simulink model "bicyclemodel_sin"  (R2021a)
settings: Solver=FixedStepAuto  StartTime=0.0  StopTime=tf  FixedStep=dt  RelTol=1e-3
values from neighbouring files (symbols this model uses):
  I = 2500    [E3_7.m]    (also in E3_8.m)
  Kf = 55000    [E3_7.m]    (also in E3_8.m = 72500)
  Kr = 60000    [E3_7.m]    (also in E3_8.m = 42500)
  lf = 1.1    [E3_7.m]    (also in E3_8.m)
  lr = 1.6    [E3_7.m]    (also in E3_8.m)
  m = 1500    [E3_7.m]    (also in E3_8.m)
  Sf = 0.04    [E3_7.m]    (also in E3_8.m; freqresponse.m = out.ScopeData.signals(1,1).values(:,1))
  V = 100/3.6    (= 27.7777777778)    [E3_7.m]    (also in E3_8.m = 38.8888888889)
settings Model: Creator=abeam  LastModifiedBy=abeam

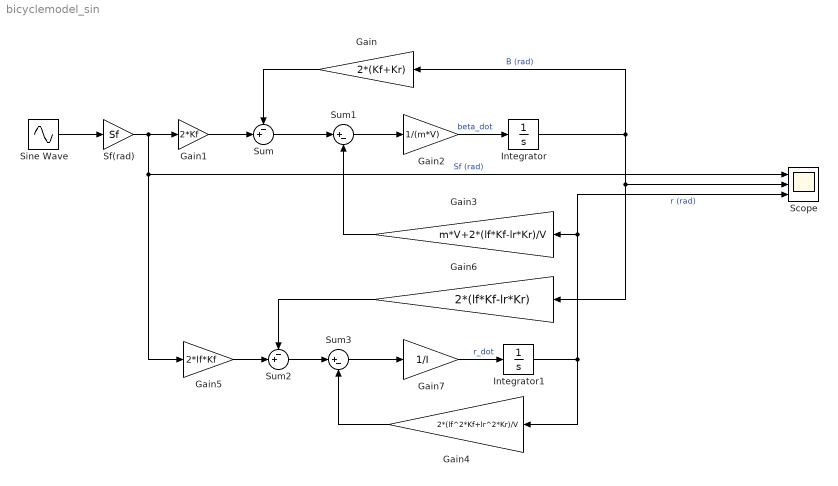
== system bicyclemodel_sin ==
  Gain : Gain  Gain=2*(Kf+Kr)
  Gain1 : Gain  Gain=2*Kf
  Gain2 : Gain  Gain=1/(m*V)
  Gain3 : Gain  Gain=m*V+2*(lf*Kf-lr*Kr)/V
  Gain4 : Gain  Gain=2*(lf^2*Kf+lr^2*Kr)/V
  Gain5 : Gain  Gain=2*lf*Kf
  Gain6 : Gain  Gain=2*(lf*Kf-lr*Kr)
  Gain7 : Gain  Gain=1/I
  Integrator : Integrator
  Integrator1 : Integrator
  Scope : Scope  NumInputPorts=3
  Sf(rad) : Gain  Gain=Sf
  Sine Wave : Sin  Amplitude=0.04  Frequency=0.5*2*pi  SampleTime=0
  Sum : Sum  Inputs=-+|
  Sum1 : Sum  Inputs=|+-
  Sum2 : Sum  Inputs=-+|
  Sum3 : Sum  Inputs=|+-
  wires:
  Sine Wave/1 -> Sf(rad)/1
  Gain1/1 -> Sum/2
  Sf(rad)/1 -> Scope/1, Gain5/1, Gain1/1  "Sf (rad)"
  Sum/1 -> Sum1/1
  Gain/1 -> Sum/1
  Sum1/1 -> Gain2/1
  Gain2/1 -> Integrator/1  "beta_dot"
  Integrator/1 -> Scope/2, Gain6/1, Gain/1  "B (rad)"
  Gain3/1 -> Sum1/2
  Gain5/1 -> Sum2/2
  Sum2/1 -> Sum3/1
  Gain6/1 -> Sum2/1
  Sum3/1 -> Gain7/1
  Gain4/1 -> Sum3/2
  Gain7/1 -> Integrator1/1  "r_dot"
  Integrator1/1 -> Scope/3, Gain3/1, Gain4/1  "r (rad)"
